simulink model "COPYBALANCEControlSystem"  (R2022a)
settings: Solver=VariableStepAuto  StartTime=0.0  StopTime=20  RelTol=1e-3
libraries: simulink x3, slpidlib x2
settings Model: Creator=ebert  LastModifiedBy=ebert

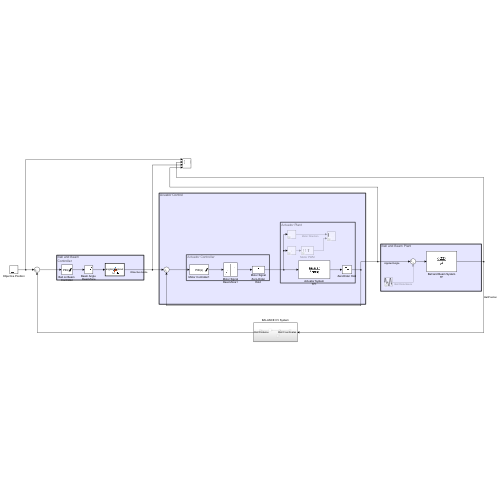
[thumbnail: Simulink's stored preview of the top-level diagram]
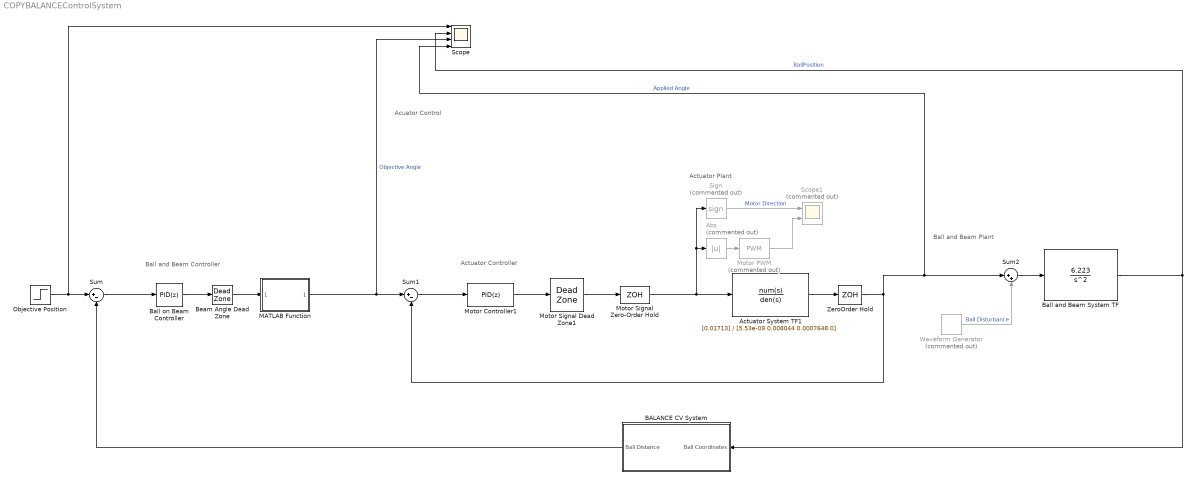
== system COPYBALANCEControlSystem ==
  note: Ball and Beam Plant
  note: Actuator Plant
  note: Actuator Controller
  note: Ball and Beam
      | Controller
  note: Acuator Control
  Abs : Abs  Commented=on  SaturateOnIntegerOverflow=off
  Actuator System TF1 : TransferFcn  Numerator=[0.01713]  Denominator=[5.53e-09 0.008044 0.0007648 0]
  BALANCE CV System : Subsystem
  Ball and Beam System TF : TransferFcn  Numerator=[6.223]  Denominator=[1 0 0]
  Ball on Beam Controller : slpidlib/PID Controller  Controller=PID  Form=Parallel  TimeDomain=Discrete-time  UseExternalTs=off  SampleTime=1/30  IntegratorMethod=Forward Euler  FilterMethod=Forward Euler  ControllerParametersSource=internal  P=0.110647526065682  I=0.00984218983062414  UseKiTs=off  D=0.298180317605175  N=4.92152866164286  UseFilter=on  TunerSelectOption=Transfer Function Based (PID Tuner App)  InitialConditionSource=internal  InitialConditionForIntegrator=0  InitialConditionForFilter=0  DifferentiatorICPrevScaledInput=0  ExternalReset=none  TrackingMode=off  Kt=1  LimitOutput=on  SatLimitsSource=internal  UpperSaturationLimit=0.3  LowerSaturationLimit=-0.3  LinearizeAsGain=off  AntiWindupMode=clamping  Kb=1  POutMin=[]  POutMax=[]  IOutMin=[]  IOutMax=[]  DOutMin=[]  DOutMax=[]  NOutMin=[]  NOutMax=[]  SumOutMin=[]  SumOutMax=[]  SaturationOutMin=[]  SaturationOutMax=[]  PParamMin=[]  PParamMax=[]  IParamMin=[]  IParamMax=[]  DParamMin=[]  DParamMax=[]  NParamMin=[]  NParamMax=[]  KbParamMin=[]  KbParamMax=[]  KtParamMin=[]  KtParamMax=[]  KbOutMin=[]  KbOutMax=[]  KtOutMin=[]  KtOutMax=[]  IntegratorOutMin=[]  IntegratorOutMax=[]  FilterOutMin=[]  FilterOutMax=[]  SumI1OutMin=[]  SumI1OutMax=[]  SumI2OutMin=[]  SumI2OutMax=[]  SumI3OutMin=[]  SumI3OutMax=[]  SumI4OutMin=[]  SumI4OutMax=[]  SumDOutMin=[]  SumDOutMax=[]  DifferentiatorOutMin=[]  DifferentiatorOutMax=[]  FilterDiffOutCoefMin=[]  FilterDiffOutCoefMax=[]  ReciprocalOutMin=[]  ReciprocalOutMax=[]  SumDenOutMin=[]  SumDenOutMax=[]  SumNumOutMin=[]  SumNumOutMax=[]  DivideOutMin=[]  DivideOutMax=[]  UdiffTsProdOutMin=[]  UdiffTsProdOutMax=[]  NTsProdOutMin=[]  NTsProdOutMax=[]  UintegralTsProdOutMin=[]  UintegralTsProdOutMax=[]  UngainTsProdOutMin=[]  UngainTsProdOutMax=[]  IntegratorContinuousStateAttributes=''  IntegratorStateMustResolveToSignalObject=off  IntegratorRTWStateStorageClass=Auto  FilterContinuousStateAttributes=''  FilterStateMustResolveToSignalObject=off  FilterRTWStateStorageClass=Auto  ParallelPVariant=InternalParameters  IdealPVariant=Disabled  IVariant=InternalParameters  DVariant=InternalParameters  IntegratorVariant=Discrete  SatVariant=Enabled  AWVariant=DiscClampingParallel  PCopyVariant=Disabled  TRVariant=Disabled  FdbkBlocksVariant=Forward  IdealPFdbkVariant=Disabled  SatFdbkVariant=Disabled  DerivativeFilterVariant=ForwardEulerFilter  NVariant=InternalParameters  NCopyVariant=Disabled  FilterICVariant=InternalICsFilter  IntegratorICVariant=InternalICs  ExternalResetVariant=Disabled  TRSumVariant=Passthrough  SumFdbkVariant=Disabled  SumVariant=Sum_PID  TsampFilterVariant=InternalTs  TsampNgainVariant=Passthrough  TsampIntegralVariant=Passthrough  ExternalSaturationOutDataTypeStr=Inherit: Same as second input  aMode=0
  Beam Angle Dead Zone : DeadZone  LowerValue=-0.001  UpperValue=0.001
  MATLAB Function : MATLAB Function  TreatAsAtomicUnit=on
  Motor Controller1 : slpidlib/PID Controller  Controller=PID  Form=Parallel  TimeDomain=Discrete-time  UseExternalTs=off  SampleTime=1/30  IntegratorMethod=Forward Euler  FilterMethod=Forward Euler  ControllerParametersSource=internal  P=26.4845239685581  I=22.2987513395518  UseKiTs=off  D=7.31174263119045  N=25.5040307304801  UseFilter=on  TunerSelectOption=Transfer Function Based (PID Tuner App)  InitialConditionSource=internal  InitialConditionForIntegrator=0  InitialConditionForFilter=0  DifferentiatorICPrevScaledInput=0  ExternalReset=none  TrackingMode=off  Kt=1  LimitOutput=on  SatLimitsSource=internal  UpperSaturationLimit=0.9  LowerSaturationLimit=-0.9  LinearizeAsGain=off  AntiWindupMode=clamping  Kb=1  POutMin=[]  POutMax=[]  IOutMin=[]  IOutMax=[]  DOutMin=[]  DOutMax=[]  NOutMin=[]  NOutMax=[]  SumOutMin=[]  SumOutMax=[]  SaturationOutMin=[]  SaturationOutMax=[]  PParamMin=[]  PParamMax=[]  IParamMin=[]  IParamMax=[]  DParamMin=[]  DParamMax=[]  NParamMin=[]  NParamMax=[]  KbParamMin=[]  KbParamMax=[]  KtParamMin=[]  KtParamMax=[]  KbOutMin=[]  KbOutMax=[]  KtOutMin=[]  KtOutMax=[]  IntegratorOutMin=[]  IntegratorOutMax=[]  FilterOutMin=[]  FilterOutMax=[]  SumI1OutMin=[]  SumI1OutMax=[]  SumI2OutMin=[]  SumI2OutMax=[]  SumI3OutMin=[]  SumI3OutMax=[]  SumI4OutMin=[]  SumI4OutMax=[]  SumDOutMin=[]  SumDOutMax=[]  DifferentiatorOutMin=[]  DifferentiatorOutMax=[]  FilterDiffOutCoefMin=[]  FilterDiffOutCoefMax=[]  ReciprocalOutMin=[]  ReciprocalOutMax=[]  SumDenOutMin=[]  SumDenOutMax=[]  SumNumOutMin=[]  SumNumOutMax=[]  DivideOutMin=[]  DivideOutMax=[]  UdiffTsProdOutMin=[]  UdiffTsProdOutMax=[]  NTsProdOutMin=[]  NTsProdOutMax=[]  UintegralTsProdOutMin=[]  UintegralTsProdOutMax=[]  UngainTsProdOutMin=[]  UngainTsProdOutMax=[]  IntegratorContinuousStateAttributes=''  IntegratorStateMustResolveToSignalObject=off  IntegratorRTWStateStorageClass=Auto  FilterContinuousStateAttributes=''  FilterStateMustResolveToSignalObject=off  FilterRTWStateStorageClass=Auto  ParallelPVariant=InternalParameters  IdealPVariant=Disabled  IVariant=InternalParameters  DVariant=InternalParameters  IntegratorVariant=Discrete  SatVariant=Enabled  AWVariant=DiscClampingParallel  PCopyVariant=Disabled  TRVariant=Disabled  FdbkBlocksVariant=Forward  IdealPFdbkVariant=Disabled  SatFdbkVariant=Disabled  DerivativeFilterVariant=ForwardEulerFilter  NVariant=InternalParameters  NCopyVariant=Disabled  FilterICVariant=InternalICsFilter  IntegratorICVariant=InternalICs  ExternalResetVariant=Disabled  TRSumVariant=Passthrough  SumFdbkVariant=Disabled  SumVariant=Sum_PID  TsampFilterVariant=InternalTs  TsampNgainVariant=Passthrough  TsampIntegralVariant=Passthrough  ExternalSaturationOutDataTypeStr=Inherit: Same as second input  aMode=0
  Motor PWM : simulink/Discontinuities/PWM  Commented=on  DisableCoverage=on  Period=1  DisallowZeroDutyCycle=off  RunAtFixedTimeIntervals=off  SampleTime=0.1
  Motor Signal Dead Zone1 : DeadZone  LowerValue=-0.1  UpperValue=0.1
  "Motor Signal Zero-Order Hold " : ZeroOrderHold  SampleTime=-1
  Objective Position : Step  Time=0  After=0.173  SampleTime=0
  Scope : Scope  NumInputPorts=4
  Scope1 : Scope  Commented=on  NumInputPorts=2
  Sign : Signum  Commented=on
  Sum : Sum  Inputs=|+-
  Sum1 : Sum  Inputs=|+-
  Sum2 : Sum  Inputs=|++
  Waveform Generator : simulink/Sources/Waveform Generator  Commented=on  OutMin=[]  OutMax=[]  OutDataTypeStr=double  SelectedSignal=1  Signals=sin(0.001,3,1)  BlockNames=MultiportSwitch_d9878704260749e  SampleTime=0.1
  ZeroOrder Hold : ZeroOrderHold  SampleTime=-1
  wires:
  Objective Position/1 -> Scope/1, Sum/1
  BALANCE CV System/1(Ball Distance) -> Sum/2
  MATLAB Function/1(angleout) -> Scope/3, Sum1/1  "Objective Angle"
  Sum/1 -> Ball on Beam Controller/1
  Beam Angle Dead Zone/1 -> MATLAB Function/1(anglein)
  Ball on Beam Controller/1 -> Beam Angle Dead Zone/1
  Motor Controller1/1 -> Motor Signal Dead Zone1/1
  Motor Signal Dead Zone1/1 -> "Motor Signal Zero-Order Hold "/1
  Sum1/1 -> Motor Controller1/1
  Sign/1 -> Scope1/1  "Motor Direction"
  Motor PWM/1 -> Scope1/2
  Abs/1 -> Motor PWM/1
  "Motor Signal Zero-Order Hold "/1 -> Sign/1, Abs/1, Actuator System TF1/1
  Actuator System TF1/1 -> ZeroOrder Hold/1
  Sum2/1 -> Ball and Beam System TF/1
  Waveform Generator/1 -> Sum2/2  "Ball Disturbance"
  Ball and Beam System TF/1 -> BALANCE CV System/1(Ball Coordinates), Scope/2  "BallPosition"
  ZeroOrder Hold/1 -> Sum1/2, Scope/4, Sum2/1  "Applied Angle"

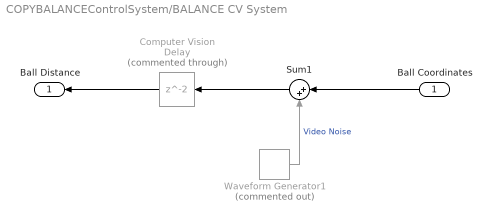
== system COPYBALANCEControlSystem/BALANCE CV System ==
  Ball Coordinates : Inport
  Computer Vision Delay : Delay  Commented=through
  Sum1 : Sum  Inputs=|++
  Waveform Generator1 : simulink/Sources/Waveform Generator  Commented=on  OutMin=[]  OutMax=[]  OutDataTypeStr=double  SelectedSignal=1  Signals=sin(0.0001,3,1)  BlockNames=MultiportSwitch_425a7e8e9f63443  SampleTime=0.1
  Ball Distance : Outport
  wires:
  Waveform Generator1/1 -> Sum1/2  "Video Noise"
  Sum1/1 -> Computer Vision Delay/1
  Computer Vision Delay/1 -> Ball Distance/1
  Ball Coordinates/1 -> Sum1/1

== matlab function COPYBALANCEControlSystem/MATLAB Function ==
  data: anglein input; angleout output
function angleout = disturb(anglein)

if(abs(anglein)<0.01 && abs(anglein)>0.001)
    angleout=sign(anglein)*0.01;
else
    angleout=anglein;
end
end
